simulink model "quad_with_sensor_fusion_discrete"  (R2022b)
settings: Solver=FixedStepDiscrete  StartTime=0.0  StopTime=120  FixedStep=0.005  RelTol=1e-3
values from neighbouring files (symbols this model uses):
  Ixc = 9373.661914436/1e6    (= 0.00937366191444)    [ParamsInit_test.m]
  Iyc = 11755.067703159/1e6    (= 0.0117550677032)    [ParamsInit_test.m]
  Izc = 17533.553367555/1e6    (= 0.0175335533676)    [ParamsInit_test.m]
  kd_h = damp_ratio_h*2*sqrt(kp_h*Vehicle.Airframe.mass)    [ParamsInit_test.m]
  kd_phi = damp_ratio_phi*2*sqrt(kp_phi*Ixc)    [ParamsInit_test.m]
  kd_theta = damp_ratio_theta*2*sqrt(kp_theta*Iyc)    [ParamsInit_test.m]
  kd_yaw = damp_ratio_yaw*2*sqrt(kp_yaw*Izc)    [ParamsInit_test.m]
  kp_h = omega_n_h^2*Vehicle.Airframe.mass    [ParamsInit_test.m]
  kp_phi = omega_n_phi^2*Ixc    (= 0.937366191444)    [ParamsInit_test.m]
  kp_position = 0.1    [ParamsInit_test.m]
  kp_theta = omega_n_theta^2*Iyc    (= 1.17550677032)    [ParamsInit_test.m]
  kp_vx = 0.25    [ParamsInit_test.m]
  kp_vy = 0.25    [ParamsInit_test.m]
  kp_yaw = omega_n_yaw^2*Izc    (= 0.0175335533676)    [ParamsInit_test.m]
undefined symbols (not defined in the file or in its folder): DiscIntNeverNeededParam, Vehicle
libraries: simulink x3, aerolibconvert2 x2, mspfiltlib x1, sensorinslib x1, aerolibasang x1, sharedtransform x1, mspsensorlib x1, sensorgpslib x1, aerolibanimutils x1, uavutilslib x1
(part 1 of 2)
settings Model: Creator=gaowe  LastModifiedBy=GMS
settings ModelReferenceCC: EnableRefExpFcnMdlSchedulingChecks=on
settings RTWCC: DLArmComputeVersion=19.05

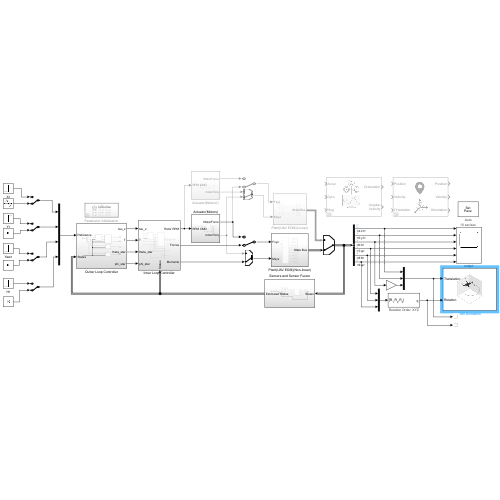
[thumbnail: Simulink's stored preview of the top-level diagram]
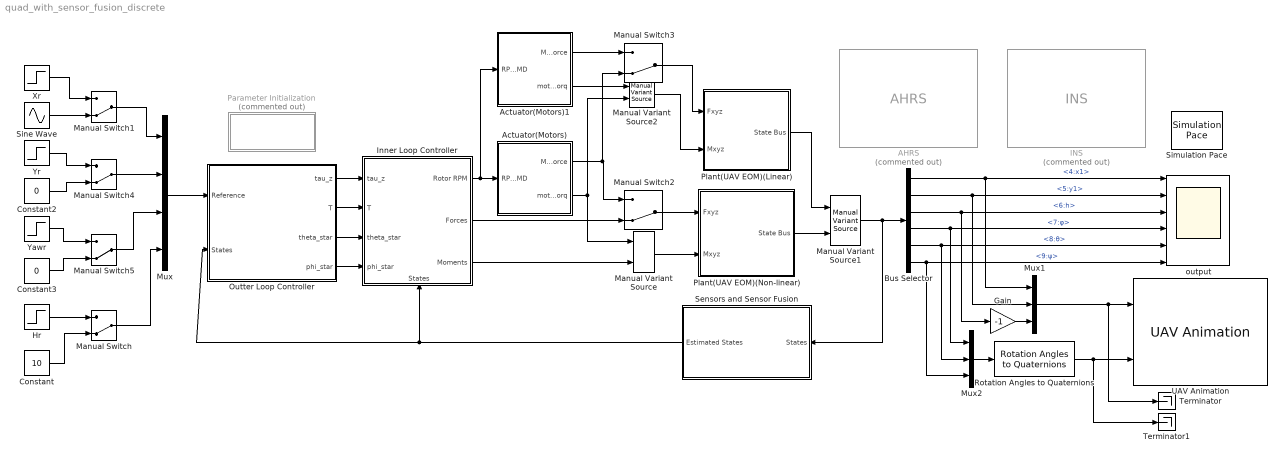
== system quad_with_sensor_fusion_discrete ==
  AHRS : mspfiltlib/AHRS  Commented=on  DispRefFrame=NED  DecimationFactor=1  InitialProcessNoise=ahrsfilter.defaultProcessNoise  OrientationFormat=quaternion  SimulateUsing=Interpreted execution  AccelerometerNoise=0.0001924722  GyroscopeNoise=9.1385e-5  MagnetometerNoise=0.1  GyroscopeDriftNoise=3.0462e-13  LinearAccelerationNoise=0.0096236100000000012  MagneticDisturbanceNoise=0.5  LinearAccelerationDecayFactor=0.5  MagneticDisturbanceDecayFactor=0.5  ExpectedMagneticFieldStrength=50
  Actuator(Motors) : Subsystem
  Actuator(Motors)1 : Subsystem
  Bus Selector : BusSelector  OutputSignals=4:x1,5:y1,6:h,7:φ,8:θ,9:ψ
  Constant : Constant  Value=10  SampleTime=0.005
  Constant2 : Constant  Value=0  SampleTime=0.005
  Constant3 : Constant  Value=0  SampleTime=0.005
  Gain : Gain  Gain=-1
  Hr : Step  Time=0  After=20  SampleTime=0.005
  INS : sensorinslib/INS  Commented=on  MountingLocation=[0 0 0]  RollAccuracy=0.2  PitchAccuracy=0.2  YawAccuracy=1  PositionAccuracy=1  VelocityAccuracy=0.05  UseAccelAndAngVel=off  AccelerationAccuracy=0  AngularVelocityAccuracy=0  TimeInput=off  PositionErrorFactor=[0 0 0]  SeedDouble=67  SimulateUsing=Interpreted execution
      settings: LibrarySourceBlock=uavsimlib/INS
  Inner Loop Controller : Subsystem
      settings: PortSchema="{\"entries\":[{\"content\":{\"sides\":[{\"content\":{\"connectorIds\":[\"In1\",\"In2\",\"In3\",\"In4\"]},\"type\":\"ConnectorPlacement.EquallySpacedRectSide\",\"uuid\":\"3024e14a-e42b-4ece-95b6-8188e577f7ea\"},{\"content\":{\"connectorIds\":[\"Out1\",\"Out2\",\"Out3\"],\"side\":\"RIGHT\"},\"type\":\"ConnectorPlacement.EquallySpacedRectSide\",\"uuid\":\"28791f10-00d9-435c-9b3a-62150bd300bc\"},{\"content\":{\"connectorIds\":[],\"side\":\"TOP\"},\"type\":\"ConnectorPlacement.EquallySpacedRectSide\",\"uuid\":\"5a81466d-668a-47df-a46c-2854fa138474\"},{\"content\":{\"connectorIds\":[\"In5\"],\"side\":\"BOTTOM\"},\"type\":\"ConnectorPlacement.EquallySpacedRectSide\",\"uuid\":\"dc01fcce-ea7b-43d7-98f8-2115160ba315\"}]},\"type\":\"ConnectorPlacement.EquallySpacedConnector\",\"uuid\":\"802a1a82-5ed7-4d3a-8fbf-5749d0aa0952\"}],\"packageUris\":[\"http://schema.mathworks.com/mf0/Connector/R2020b\"],\"version\":\"1.0\"}"
  Manual Variant Source : simulink/Signal Routing/Manual Variant Source  NumChoices=2  LabelModeActiveChoice=V_2
  Manual Variant Source1 : simulink/Signal Routing/Manual Variant Source  NumChoices=2  LabelModeActiveChoice=V_2
  Manual Variant Source2 : simulink/Signal Routing/Manual Variant Source  NumChoices=2  LabelModeActiveChoice=V_2
  Manual Switch{,1..5} (6 alike) : ManualSwitch  CurrentSetting=0
  Mux : Mux
  Mux1 : Mux  Inputs=3
  Mux2 : Mux  Inputs=3
  Outter Loop Controller : Subsystem
  Parameter Initialization : Subsystem  Commented=on  TreatAsAtomicUnit=on
  Plant(UAV EOM)(Linear) : Subsystem
  Plant(UAV EOM)(Non-linear) : Subsystem
  Rotation Angles to Quaternions : sharedtransform/Rotation Angles to Quaternions  rotationOrder=XYZ  aMode=aMode
  Sensors and Sensor Fusion : Subsystem
  Simulation Pace : aerolibanimutils/Simulation Pace  SimulationPace=10  SleepMode=Auto  OutputPaceError=off  SampleTime=1/100
  Sine Wave : Sin  SineType=Sample based  Amplitude=10  Frequency=2*pi/60  Samples=12000  SampleTime=0.005
  Terminator : Terminator
  Terminator1 : Terminator
  UAV Animation : uavutilslib/UAV Animation  UAVType=Multirotor  UAVSize=1  InertialZDirection=Down  SampleTime=0.005
  Xr : Step  Time=0  After=10  SampleTime=0.005
  Yawr : Step  Time=0  After=pi/2  SampleTime=0.005
  Yr : Step  Time=0  After=10  SampleTime=0.005
  output : Scope  NumInputPorts=6
  wires:
  Manual Variant Source1/1 -> Sensors and Sensor Fusion/1(States), Bus Selector/1
  Mux/1 -> Outter Loop Controller/1(Reference)
  Manual Switch1/1 -> Mux/1
  Constant2/1 -> Manual Switch4/2
  Yawr/1 -> Manual Switch5/1
  Hr/1 -> Manual Switch/1
  Outter Loop Controller/3(theta_star) -> Inner Loop Controller/3(theta_star)
  Outter Loop Controller/1(tau_z) -> Inner Loop Controller/1(tau_z)
  Outter Loop Controller/2(T) -> Inner Loop Controller/2(T)
  Outter Loop Controller/4(phi_star) -> Inner Loop Controller/4(phi_star)
  Inner Loop Controller/1(Rotor RPM) -> Actuator(Motors)1/1(RPM CMD), Actuator(Motors)/1(RPM CMD)
  Actuator(Motors)/1(MotorForce) -> Manual Switch3/2, Manual Switch2/1
  Actuator(Motors)/2(motorTorq) -> Manual Variant Source2/2, Manual Variant Source/1
  Bus Selector/1 -> Mux1/1, output/1  "<4:x1>"
  Bus Selector/2 -> Mux1/2, output/2  "<5:y1>"
  Bus Selector/3 -> Gain/1, output/3  "<6:h>"
  Bus Selector/4 -> Mux2/1, output/4  "<7:φ>"
  Bus Selector/5 -> Mux2/2, output/5  "<8:θ>"
  Bus Selector/6 -> Mux2/3, output/6  "<9:ψ>"
  Manual Switch/1 -> Mux/4
  Constant/1 -> Manual Switch/2
  Sine Wave/1 -> Manual Switch1/2
  Xr/1 -> Manual Switch1/1
  Inner Loop Controller/2(Forces) -> Manual Switch2/2
  Inner Loop Controller/3(Moments) -> Manual Variant Source/2
  Plant(UAV EOM)(Linear)/1(State Bus) -> Manual Variant Source1/1
  Manual Variant Source/1 -> Plant(UAV EOM)(Non-linear)/2(Mxyz)
  Manual Switch2/1 -> Plant(UAV EOM)(Non-linear)/1(Fxyz)
  Plant(UAV EOM)(Non-linear)/1(State Bus) -> Manual Variant Source1/2
  Actuator(Motors)1/1(MotorForce) -> Manual Switch3/1
  Actuator(Motors)1/2(motorTorq) -> Manual Variant Source2/1
  Manual Switch3/1 -> Plant(UAV EOM)(Linear)/1(Fxyz)
  Manual Variant Source2/1 -> Plant(UAV EOM)(Linear)/2(Mxyz)
  Manual Switch4/1 -> Mux/2
  Yr/1 -> Manual Switch4/1
  Constant3/1 -> Manual Switch5/2
  Manual Switch5/1 -> Mux/3
  Mux1/1 -> Terminator/1, UAV Animation/1
  Rotation Angles to Quaternions/1 -> Terminator1/1, UAV Animation/2
  Mux2/1 -> Rotation Angles to Quaternions/1
  Gain/1 -> Mux1/3
  Sensors and Sensor Fusion/1(Estimated States) -> Outter Loop Controller/2(States), Inner Loop Controller/5(States)

== system quad_with_sensor_fusion_discrete/Actuator(Motors) ==
  RPM CMD : Inport
  -k_T : Gain  Gain=-1.097e-5
  D4 : Constant  Value=0  SampleTime=0.005
  D5 : Constant  Value=0  SampleTime=0.005
  Mux4 : Mux  Inputs=3
  Propeller Model : MATLAB Function  TreatAsAtomicUnit=on
  Square : Math  Operator=square
  Sum of Elements : Sum  Inputs=+
  k_tau : Gain  Gain=1.779e-07
  rpm2rads : Gain  Gain=pi/30
  MotorForce : Outport
  motorTorq : Outport  Port=2
  wires:
  k_tau/1 -> motorTorq/1
  Mux4/1 -> MotorForce/1
  Sum of Elements/1 -> Mux4/3
  -k_T/1 -> Sum of Elements/1
  Square/1 -> -k_T/1, Propeller Model/1(F)
  Propeller Model/1(Mb_xy) -> k_tau/1
  D4/1 -> Mux4/1
  D5/1 -> Mux4/2
  RPM CMD/1 -> rpm2rads/1
  rpm2rads/1 -> Square/1

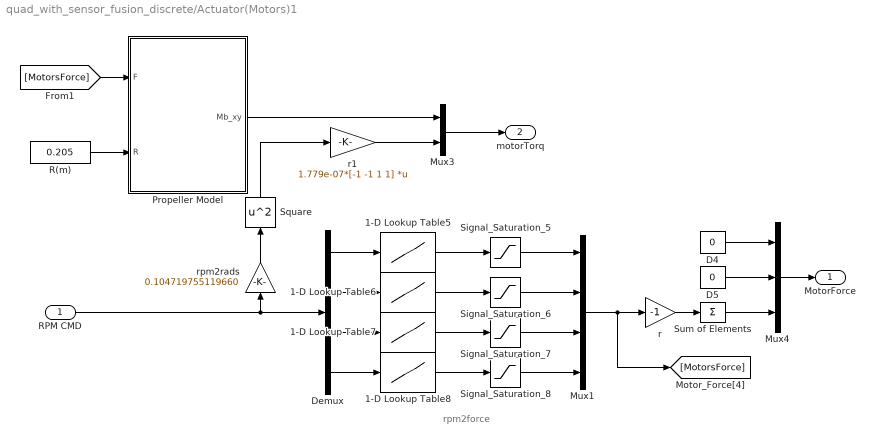
== system quad_with_sensor_fusion_discrete/Actuator(Motors)1 ==
  note: rpm2force
  RPM CMD : Inport
  1-D Lookup Table5 : Lookup_n-D  NumberOfTableDimensions=1  BreakpointsForDimension1=|  BeginIndexSearchUsingPreviousIndexResult=on  Table=|  InternalRulePriority=Speed  RndMeth=Simplest
      BreakpointsForDimension1=|
      | [2847
      | 3689
      | 4585
      | 5400
      | 6400
      | 7000
      | 7800
      | 8222
      | 9300
      | 10700]
      Table=|
      | [0.6664
      | 1.4308
      | 2.3422
      | 3.3418
      | 4.9098
      | 5.929
      | 7.399
      | 7.6244
      | 10.976
      | 13.72]
  1-D Lookup Table6 : Lookup_n-D  NumberOfTableDimensions=1  BreakpointsForDimension1=|  BeginIndexSearchUsingPreviousIndexResult=on  Table=|  InternalRulePriority=Speed  RndMeth=Simplest
      BreakpointsForDimension1=|
      | [2847
      | 3689
      | 4585
      | 5400
      | 6400
      | 7000
      | 7800
      | 8222
      | 9300
      | 10700]
      Table=|
      | [0.6664
      | 1.4308
      | 2.3422
      | 3.3418
      | 4.9098
      | 5.929
      | 7.399
      | 7.6244
      | 10.976
      | 13.72]
  1-D Lookup Table7 : Lookup_n-D  NumberOfTableDimensions=1  BreakpointsForDimension1=|  BeginIndexSearchUsingPreviousIndexResult=on  Table=|  InternalRulePriority=Speed  RndMeth=Simplest
      BreakpointsForDimension1=|
      | [2847
      | 3689
      | 4585
      | 5400
      | 6400
      | 7000
      | 7800
      | 8222
      | 9300
      | 10700]
      Table=|
      | [0.6664
      | 1.4308
      | 2.3422
      | 3.3418
      | 4.9098
      | 5.929
      | 7.399
      | 7.6244
      | 10.976
      | 13.72]
  1-D Lookup Table8 : Lookup_n-D  NumberOfTableDimensions=1  BreakpointsForDimension1=|  BeginIndexSearchUsingPreviousIndexResult=on  Table=|  InternalRulePriority=Speed  RndMeth=Simplest
      BreakpointsForDimension1=|
      | [2847
      | 3689
      | 4585
      | 5400
      | 6400
      | 7000
      | 7800
      | 8222
      | 9300
      | 10700]
      Table=|
      | [0.6664
      | 1.4308
      | 2.3422
      | 3.3418
      | 4.9098
      | 5.929
      | 7.399
      | 7.6244
      | 10.976
      | 13.72]
  D4 : Constant  Value=0
  D5 : Constant  Value=0
  Demux : Demux
  Mux1 : Mux
  Mux3 : Mux  Inputs=[2 1]
  Mux4 : Mux  Inputs=3
  Propeller Model : MATLAB Function  TreatAsAtomicUnit=on
  R(m) : Constant  Value=0.205
  Signal_Saturation_{5..8} (4 alike) : Saturate  UpperLimit=1.4*9.8  LowerLimit=0
  Square : Math  Operator=square
  Sum of Elements : Sum  Inputs=+
  r : Gain  Gain=-1
  r1 : Gain  Gain=1.779e-07*[-1 -1 1 1]  Multiplication=Matrix(K*u)
  rpm2rads : Gain  Gain=0.104719755119660
  MotorForce : Outport
  motorTorq : Outport  Port=2
  wires:
  Signal_Saturation_6/1 -> Mux1/2
  1-D Lookup Table7/1 -> Signal_Saturation_7/1
  Mux3/1 -> motorTorq/1
  1-D Lookup Table6/1 -> Signal_Saturation_6/1
  Mux4/1 -> MotorForce/1
  r1/1 -> Mux3/2
  Sum of Elements/1 -> Mux4/3
  r/1 -> Sum of Elements/1
  Mux1/1 -> [MotorsForce], r/1
  Demux/1 -> 1-D Lookup Table5/1
  Square/1 -> r1/1
  1-D Lookup Table5/1 -> Signal_Saturation_5/1
  Demux/3 -> 1-D Lookup Table7/1
  Signal_Saturation_5/1 -> Mux1/1
  1-D Lookup Table8/1 -> Signal_Saturation_8/1
  [MotorsForce] -> Propeller Model/1(F)
  Demux/4 -> 1-D Lookup Table8/1
  Demux/2 -> 1-D Lookup Table6/1
  Signal_Saturation_7/1 -> Mux1/3
  Propeller Model/1(Mb_xy) -> Mux3/1
  Signal_Saturation_8/1 -> Mux1/4
  R(m)/1 -> Propeller Model/2(R)
  D4/1 -> Mux4/1
  D5/1 -> Mux4/2
  RPM CMD/1 -> Demux/1, rpm2rads/1
  rpm2rads/1 -> Square/1

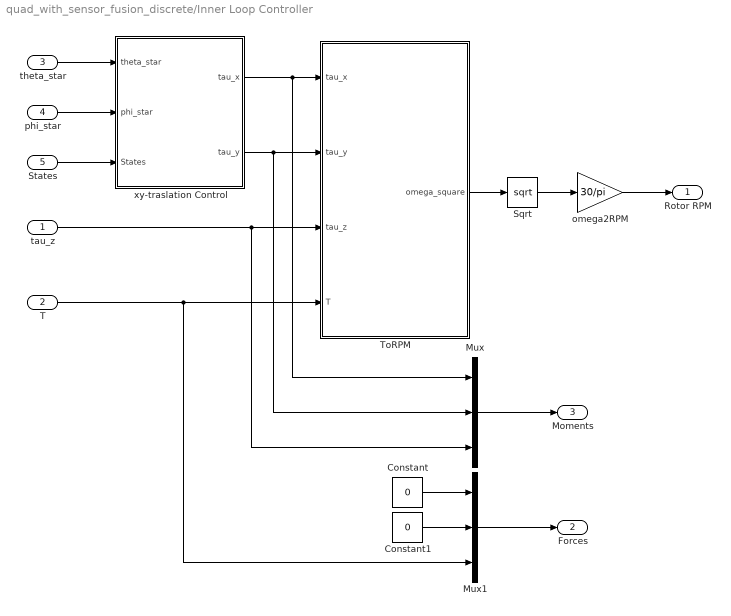
== system quad_with_sensor_fusion_discrete/Inner Loop Controller ==
  tau_z : Inport
  T : Inport  Port=2
  theta_star : Inport  Port=3
  phi_star : Inport  Port=4
  States : Inport  Port=5
  Constant : Constant  Value=0  SampleTime=0.005
  Constant1 : Constant  Value=0  SampleTime=0.005
  Mux : Mux  Inputs=3
  Mux1 : Mux  Inputs=3
  Sqrt : Sqrt
  ToRPM : MATLAB Function  TreatAsAtomicUnit=on
  omega2RPM : Gain  Gain=30/pi
  xy-traslation Control : Subsystem
  Rotor RPM : Outport
  Forces : Outport  Port=2
  Moments : Outport  Port=3
  wires:
  theta_star/1 -> xy-traslation Control/1(theta_star)
  States/1 -> xy-traslation Control/3(States)
  phi_star/1 -> xy-traslation Control/2(phi_star)
  tau_z/1 -> Mux/3, ToRPM/3(tau_z)
  xy-traslation Control/2(tau_y) -> Mux/2, ToRPM/2(tau_y)
  xy-traslation Control/1(tau_x) -> Mux/1, ToRPM/1(tau_x)
  Sqrt/1 -> omega2RPM/1
  omega2RPM/1 -> Rotor RPM/1
  ToRPM/1(omega_square) -> Sqrt/1
  Mux/1 -> Moments/1
  Constant/1 -> Mux1/1
  Constant1/1 -> Mux1/2
  Mux1/1 -> Forces/1
  T/1 -> Mux1/3, ToRPM/4(T)

== system quad_with_sensor_fusion_discrete/Outter Loop Controller ==
  Reference : Inport
  States : Inport  Port=2
  Demux : Demux
  Height Control : Subsystem
  Position Control : Subsystem
  Velocity Control : Subsystem
  Yaw Control : Subsystem
  tau_z : Outport
  T : Outport  Port=2
  theta_star : Outport  Port=3
  phi_star : Outport  Port=4
  wires:
  Reference/1 -> Demux/1
  States/1 -> Position Control/3(States), Velocity Control/3(States), Yaw Control/2(States), Height Control/2(States)
  Velocity Control/1(theta_star) -> theta_star/1
  Demux/4 -> Height Control/1(Hr)  "Hr"
  Demux/3 -> Yaw Control/1(Yawr)  "Yawr"
  Demux/2 -> Position Control/2(yr)  "Yr"
  Demux/1 -> Position Control/1(xr)  "Xr"
  Height Control/1(T) -> T/1
  Yaw Control/1(tau_z) -> tau_z/1
  Velocity Control/2(phi_star) -> phi_star/1
  Position Control/1(vxr) -> Velocity Control/1(vxr)
  Position Control/2(vyr) -> Velocity Control/2(vyr)

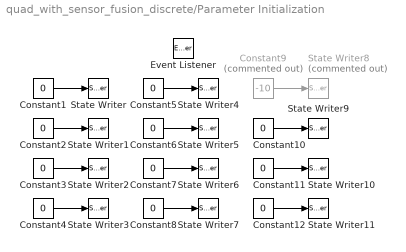
== system quad_with_sensor_fusion_discrete/Parameter Initialization ==
  Constant{1..8,10..12} (11 alike) : Constant  Value=0
  Constant9 : Constant  Commented=on  Value=-10
  Event Listener : EventListener  DisableCoverage=on  EventName=reset
  State Writer{,1..7,9..11} (11 alike) : StateWriter
  State Writer8 : StateWriter  Commented=on
  wires:
  Constant1/1 -> State Writer/1
  Constant2/1 -> State Writer1/1
  Constant4/1 -> State Writer3/1
  Constant3/1 -> State Writer2/1
  Constant6/1 -> State Writer5/1
  Constant7/1 -> State Writer6/1
  Constant5/1 -> State Writer4/1
  Constant8/1 -> State Writer7/1
  Constant10/1 -> State Writer9/1
  Constant11/1 -> State Writer10/1
  Constant9/1 -> State Writer8/1
  Constant12/1 -> State Writer11/1

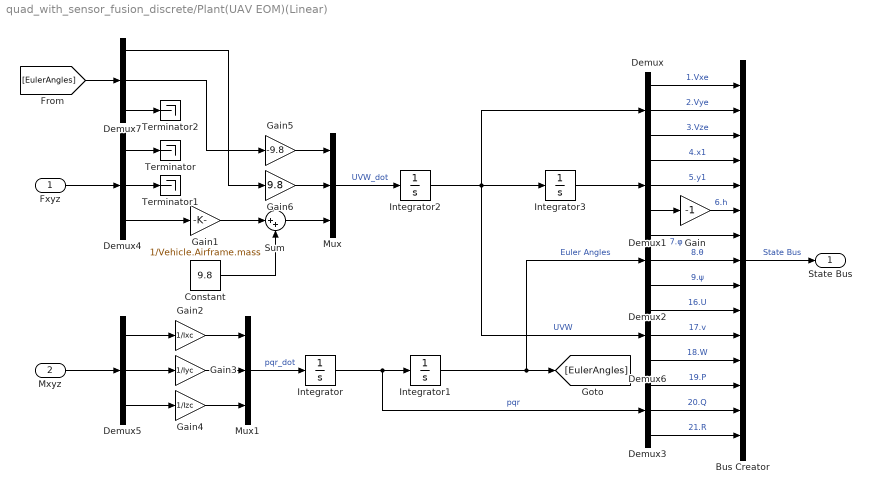
== system quad_with_sensor_fusion_discrete/Plant(UAV EOM)(Linear) ==
  Fxyz : Inport
  Mxyz : Inport  Port=2
  Bus Creator : BusCreator  Inputs=15
  Constant : Constant  Value=9.8
  Demux{,1..7} (8 alike) : Demux  Outputs=3
  Gain : Gain  Gain=-1
  Gain1 : Gain  Gain=1/Vehicle.Airframe.mass
  Gain2 : Gain  Gain=1/Ixc
  Gain3 : Gain  Gain=1/Iyc
  Gain4 : Gain  Gain=1/Izc
  Gain5 : Gain  Gain=-9.8
  Gain6 : Gain  Gain=9.8
  Integrator : Integrator  InitialCondition=[0,0,0]
  Integrator1 : Integrator  InitialCondition=[0,0,0]
  Integrator2 : Integrator  InitialCondition=[0,0,0]
  Integrator3 : Integrator  InitialCondition=[0,0,-10]
  Mux : Mux  Inputs=3
  Mux1 : Mux  Inputs=3
  Sum : Sum  Inputs=|++
  Terminator : Terminator
  Terminator1 : Terminator
  Terminator2 : Terminator
  State Bus : Outport
  wires:
  Gain/1 -> Bus Creator/6  "6.h"
  Demux/1 -> Bus Creator/1  "1.Vxe"
  Demux6/2 -> Bus Creator/11  "17.v"
  Demux3/3 -> Bus Creator/15  "21.R"
  Demux3/1 -> Bus Creator/13  "19.P"
  Demux6/1 -> Bus Creator/10  "16.U"
  Demux2/2 -> Bus Creator/8  "8.θ"
  Demux2/1 -> Bus Creator/7  "7.φ"
  Demux1/3 -> Gain/1
  Demux2/3 -> Bus Creator/9  "9.ψ"
  Demux1/2 -> Bus Creator/5  "5.y1"
  Demux3/2 -> Bus Creator/14  "20.Q"
  Demux6/3 -> Bus Creator/12  "18.W"
  Demux/3 -> Bus Creator/3  "3.Vze"
  Demux1/1 -> Bus Creator/4  "4.x1"
  Demux/2 -> Bus Creator/2  "2.Vye"
  Bus Creator/1 -> State Bus/1  "State Bus"
  Fxyz/1 -> Demux4/1
  Mxyz/1 -> Demux5/1
  Demux4/1 -> Terminator/1
  Demux4/2 -> Terminator1/1
  Demux4/3 -> Gain1/1
  Gain1/1 -> Sum/1
  Demux5/2 -> Gain3/1
  Demux5/1 -> Gain2/1
  Demux5/3 -> Gain4/1
  Mux1/1 -> Integrator/1  "pqr_dot"
  Gain3/1 -> Mux1/2
  Gain2/1 -> Mux1/1
  Gain4/1 -> Mux1/3
  Integrator/1 -> Demux3/1, Integrator1/1  "pqr"
  Integrator1/1 -> [EulerAngles], Demux2/1  "Euler Angles"
  Gain5/1 -> Mux/1
  [EulerAngles] -> Demux7/1
  Demux7/1 -> Gain6/1
  Demux7/2 -> Gain5/1
  Gain6/1 -> Mux/2
  Demux7/3 -> Terminator2/1
  Mux/1 -> Integrator2/1  "UVW_dot"
  Integrator2/1 -> Demux/1, Integrator3/1, Demux6/1  "UVW"
  Integrator3/1 -> Demux1/1
  Constant/1 -> Sum/2
  Sum/1 -> Mux/3

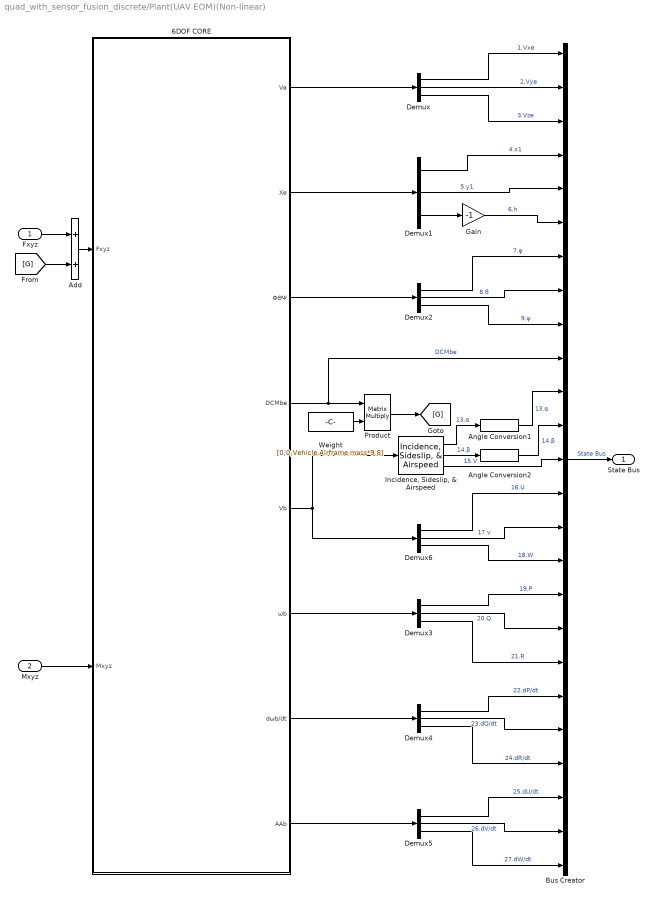
== system quad_with_sensor_fusion_discrete/Plant(UAV EOM)(Non-linear) ==
  Fxyz : Inport
  Mxyz : Inport  Port=2
  6DOF CORE : Subsystem
  Add : Sum
  Angle Conversion1 : aerolibconvert2/Angle Conversion  IU=rad  OU=deg
  Angle Conversion2 : aerolibconvert2/Angle Conversion  IU=rad  OU=deg
  Bus Creator : BusCreator  Inputs=25
  Demux{,1..6} (7 alike) : Demux  Outputs=3
  Gain : Gain  Gain=-1
  "Incidence, Sideslip, & Airspeed" : aerolibasang/Incidence, Sideslip, & Airspeed
  Product : Product  Multiplication=Matrix(*)
  Weight : Constant  Value=[0;0;Vehicle.Airframe.mass*9.8]  VectorParams1D=off  SampleTime=0.005
  State Bus : Outport
  wires:
  Gain/1 -> Bus Creator/6  "6.h"
  6DOF CORE/5(Vb) -> "Incidence, Sideslip, & Airspeed"/1, Demux6/1
  6DOF CORE/1(Ve) -> Demux/1
  Demux/1 -> Bus Creator/1  "1.Vxe"
  Demux6/2 -> Bus Creator/15  "17.v"
  6DOF CORE/3(ΦΘΨ) -> Demux2/1
  Demux3/3 -> Bus Creator/19  "21.R"
  Demux5/3 -> Bus Creator/25  "27.dW/dt"
  Demux4/3 -> Bus Creator/22  "24.dR/dt"
  "Incidence, Sideslip, & Airspeed"/3 -> Bus Creator/13  "15.V"
  Demux3/1 -> Bus Creator/17  "19.P"
  Demux6/1 -> Bus Creator/14  "16.U"
  6DOF CORE/7(dωb/dt) -> Demux4/1
  Demux2/2 -> Bus Creator/8  "8.θ"
  Demux2/1 -> Bus Creator/7  "7.φ"
  "Incidence, Sideslip, & Airspeed"/1 -> Angle Conversion1/1  "13.α"
  6DOF CORE/6(ωb) -> Demux3/1
  Demux1/3 -> Gain/1
  6DOF CORE/2(Xe) -> Demux1/1
  Demux2/3 -> Bus Creator/9  "9.ψ"
  Demux4/2 -> Bus Creator/21  "23.dQ/dt"
  Demux5/2 -> Bus Creator/24  "26.dV/dt"
  Demux1/2 -> Bus Creator/5  "5.y1"
  Demux3/2 -> Bus Creator/18  "20.Q"
  Angle Conversion2/1 -> Bus Creator/12  "14.β"
  Demux5/1 -> Bus Creator/23  "25.dU/dt"
  Demux6/3 -> Bus Creator/16  "18.W"
  6DOF CORE/8(AAb) -> Demux5/1
  Demux4/1 -> Bus Creator/20  "22.dP/dt"
  Angle Conversion1/1 -> Bus Creator/11  "13.α"
  Demux/3 -> Bus Creator/3  "3.Vze"
  "Incidence, Sideslip, & Airspeed"/2 -> Angle Conversion2/1  "14.β"
  Demux1/1 -> Bus Creator/4  "4.x1"
  Demux/2 -> Bus Creator/2  "2.Vye"
  Bus Creator/1 -> State Bus/1  "State Bus"
  Fxyz/1 -> Add/1
  Mxyz/1 -> 6DOF CORE/2(Mxyz)
  Product/1 -> [G]
  Weight/1 -> Product/2
  6DOF CORE/4(DCMbe) -> Bus Creator/10, Product/1  "DCMbe"
  [G] -> Add/2
  Add/1 -> 6DOF CORE/1(Fxyz)

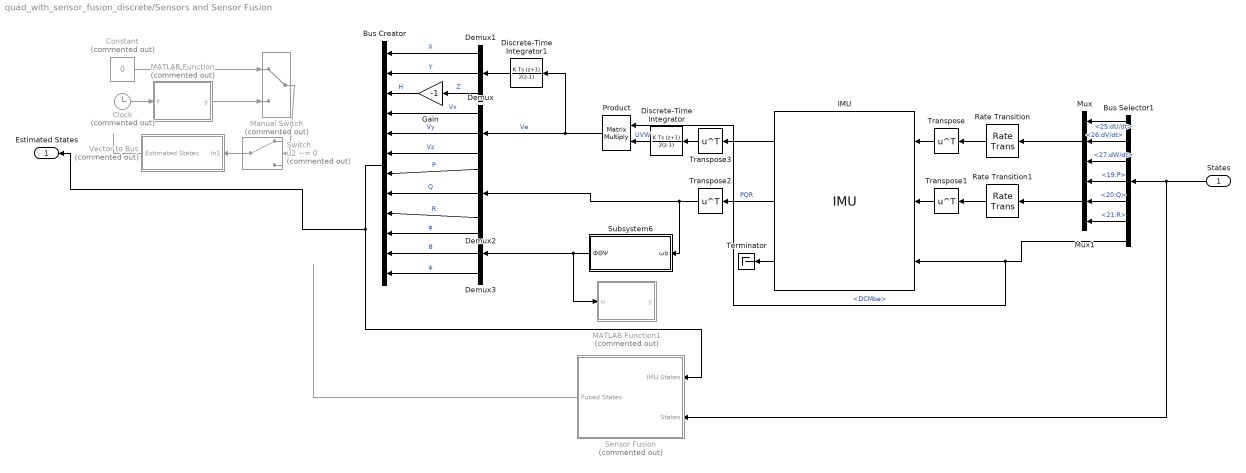
== system quad_with_sensor_fusion_discrete/Sensors and Sensor Fusion ==
  States : Inport
  Bus Creator : BusCreator  Inputs=12
  Bus Selector1 : BusSelector  OutputSignals=25:dU/dt,26:dV/dt,27:dW/dt,19:P,20:Q,21:R,DCMbe
  Clock : Clock  Commented=on
  Constant : Constant  Commented=on  Value=0  SampleTime=0.005
  Demux{,1..3} (4 alike) : Demux  Outputs=3
  Discrete-Time Integrator : DiscreteIntegrator  IntegratorMethod=Integration: Trapezoidal  SampleTime=0.005  ICPrevOutput=DiscIntNeverNeededParam  ICPrevScaledInput=DiscIntNeverNeededParam
  Discrete-Time Integrator1 : DiscreteIntegrator  IntegratorMethod=Integration: Trapezoidal  SampleTime=0.005  ICPrevOutput=DiscIntNeverNeededParam  ICPrevScaledInput=DiscIntNeverNeededParam
  Gain : Gain  Gain=-1
  IMU : mspsensorlib/IMU  DispRefFrame=NED  Temperature=25  MagneticFieldNED=[ 27.5550, -2.4169, -16.0849 ]  MagneticFieldENU=[ -2.4169, 27.5550, 16.0849 ]  SeedDouble=67  SimulateUsing=Interpreted execution  AccelParamsMeasurementRange=19.613  AccelParamsResolution=0.0023928  AccelParamsConstantBias=[ 0, 0, 0 ]  AccelParamsAxesMisalignment=[0 0 0]  AccelParamsNoiseDensity=0.01*ones(1,3)  AccelParamsBiasInstability=[ 0, 0, 0 ]  AccelParamsRandomWalk=[ 0, 0, 0 ]  AccelParamsTemperatureBias=[ 0, 0, 0 ]  AccelParamsTemperatureScaleFactor=[ 0, 0, 0 ]  GyroParamsMeasurementRange=4.3633  GyroParamsResolution=0.0011  GyroParamsConstantBias=[ 0, 0, 0 ]  GyroParamsAxesMisalignment=0  GyroParamsAccelerationBias=[ 0, 0, 0 ]  GyroParamsNoiseDensity=1e-3*ones(1,3)  GyroParamsBiasInstability=[ 0, 0, 0 ]  GyroParamsRandomWalk=[ 0, 0, 0 ]  GyroParamsTemperatureBias=[ 0, 0, 0 ]  GyroParamsTemperatureScaleFactor=[ 0, 0, 0 ]  MagParamsMeasurementRange=1000  MagParamsResolution=0.1  MagParamsConstantBias=[ 0, 0, 0 ]  MagParamsAxesMisalignment=[0 0 0]  MagParamsNoiseDensity=[0.0424 0.0424 0.0424]  MagParamsBiasInstability=[ 0, 0, 0 ]  MagParamsRandomWalk=[ 0, 0, 0 ]  MagParamsTemperatureBias=[ 0, 0, 0 ]  MagParamsTemperatureScaleFactor=[ 0, 0, 0 ]
  MATLAB Function : MATLAB Function  Commented=on  TreatAsAtomicUnit=on
  MATLAB Function1 : MATLAB Function  Commented=on  TreatAsAtomicUnit=on
  Manual Switch : ManualSwitch  Commented=on
  Mux : Mux  Inputs=3
  Mux1 : Mux  Inputs=3
  Product : Product  Multiplication=Matrix(*)
  Rate Transition : RateTransition
  Rate Transition1 : RateTransition
  Sensor Fusion : Subsystem  Commented=on
  Subsystem6 : Subsystem
  Switch : Switch  Commented=on  Criteria=u2 ~= 0  SaturateOnIntegerOverflow=off  InputSameDT=off
  Terminator : Terminator
  Transpose{,1..3} (4 alike) : Math  Operator=transpose
  Vector to Bus : Subsystem  Commented=on
  Estimated States : Outport
  wires:
  Bus Creator/1 -> Estimated States/1, Sensor Fusion/1(IMU States)
  States/1 -> Sensor Fusion/2(States), Bus Selector1/1
  Subsystem6/1(ΦΘΨ) -> MATLAB Function1/1(u), Demux3/1
  Bus Selector1/4 -> Mux1/1  "<19:P>"
  Bus Selector1/5 -> Mux1/2  "<20:Q>"
  Bus Selector1/6 -> Mux1/3  "<21:R>"
  Bus Selector1/1 -> Mux/1  "<25:dU/dt>"
  Bus Selector1/2 -> Mux/2  "<26:dV/dt>"
  Bus Selector1/3 -> Mux/3  "<27:dW/dt>"
  Clock/1 -> MATLAB Function/1(t)
  MATLAB Function/1(y) -> Manual Switch/2
  IMU/3 -> Terminator/1
  IMU/1 -> Transpose3/1
  IMU/2 -> Transpose2/1  "PQR"
  Discrete-Time Integrator/1 -> Product/2  "UVW"
  Product/1 -> Discrete-Time Integrator1/1, Demux/1  "Ve"
  Demux/1 -> Bus Creator/4  "Vx"
  Demux/2 -> Bus Creator/5  "Vy"
  Demux/3 -> Bus Creator/6  "Vz"
  Discrete-Time Integrator1/1 -> Demux1/1
  Demux1/1 -> Bus Creator/1  "X"
  Demux1/2 -> Bus Creator/2  "Y"
  Demux1/3 -> Gain/1  "Z"
  Gain/1 -> Bus Creator/3  "H"
  Demux2/1 -> Bus Creator/7  "P"
  Demux2/2 -> Bus Creator/8  "Q"
  Demux2/3 -> Bus Creator/9  "R"
  Demux3/1 -> Bus Creator/10  "φ"
  Demux3/2 -> Bus Creator/11  "θ"
  Demux3/3 -> Bus Creator/12  "ψ"
  Bus Selector1/7 -> Product/1, IMU/3  "<DCMbe>"
  Sensor Fusion/1(Fused States) -> ?
  Vector to Bus/1(Estimated States) -> ?
  Constant/1 -> Manual Switch/1
  Manual Switch/1 -> Switch/2
  Switch/1 -> Vector to Bus/1(In1)
  Transpose/1 -> IMU/1
  Transpose1/1 -> IMU/2
  Mux/1 -> Rate Transition/1
  Mux1/1 -> Rate Transition1/1
  Rate Transition/1 -> Transpose/1
  Rate Transition1/1 -> Transpose1/1
  Transpose2/1 -> Subsystem6/1(ωb), Demux2/1
  Transpose3/1 -> Discrete-Time Integrator/1

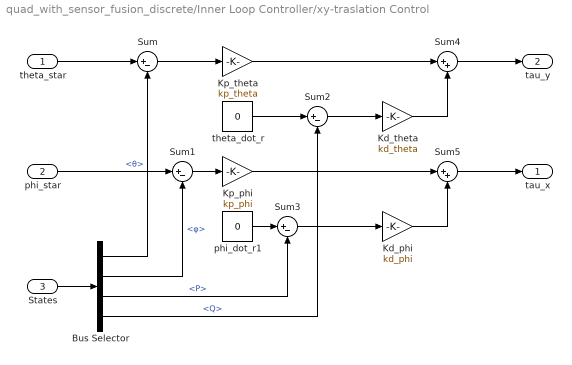
== system quad_with_sensor_fusion_discrete/Inner Loop Controller/xy-traslation Control ==
  theta_star : Inport
  phi_star : Inport  Port=2
  States : Inport  Port=3
  Bus Selector : BusSelector  OutputSignals=θ,φ,P,Q
  Kd_phi : Gain  Gain=kd_phi
  Kd_theta : Gain  Gain=kd_theta
  Kp_phi : Gain  Gain=kp_phi
  Kp_theta : Gain  Gain=kp_theta
  Sum{,1..3} (4 alike) : Sum  Inputs=|+-
  Sum4 : Sum  Inputs=|++
  Sum5 : Sum  Inputs=|++
  phi_dot_r1 : Constant  Value=0  SampleTime=0.005
  theta_dot_r : Constant  Value=0  SampleTime=0.005
  tau_x : Outport
  tau_y : Outport  Port=2
  wires:
  theta_star/1 -> Sum/1
  States/1 -> Bus Selector/1
  Bus Selector/1 -> Sum/2  "<θ>"
  phi_star/1 -> Sum1/1
  Bus Selector/2 -> Sum1/2  "<φ>"
  Sum/1 -> Kp_theta/1
  Sum1/1 -> Kp_phi/1
  Bus Selector/3 -> Sum3/2  "<P>"
  Bus Selector/4 -> Sum2/2  "<Q>"
  Kp_theta/1 -> Sum4/1
  theta_dot_r/1 -> Sum2/1
  Kp_phi/1 -> Sum5/1
  Sum2/1 -> Kd_theta/1
  Kd_theta/1 -> Sum4/2
  Sum4/1 -> tau_y/1
  phi_dot_r1/1 -> Sum3/1
  Sum3/1 -> Kd_phi/1
  Sum5/1 -> tau_x/1
  Kd_phi/1 -> Sum5/2

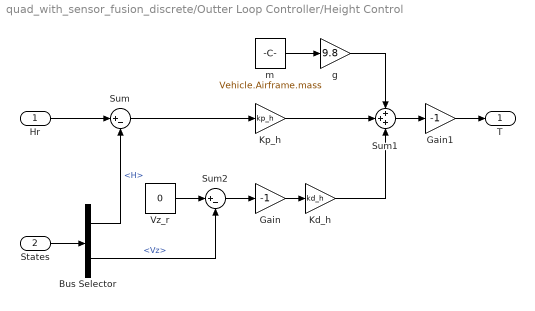
== system quad_with_sensor_fusion_discrete/Outter Loop Controller/Height Control ==
  Hr : Inport
  States : Inport  Port=2
  Bus Selector : BusSelector  OutputSignals=H,Vz
  Gain : Gain  Gain=-1
  Gain1 : Gain  Gain=-1
  Kd_h : Gain  Gain=kd_h
  Kp_h : Gain  Gain=kp_h
  Sum : Sum  Inputs=|+-
  Sum1 : Sum  Inputs=+++
  Sum2 : Sum  Inputs=|+-
  Vz_r : Constant  Value=0  SampleTime=0.005
  g : Gain  Gain=9.8
  m : Constant  Value=Vehicle.Airframe.mass  SampleTime=0.005
  T : Outport
  wires:
  Sum1/1 -> Gain1/1
  States/1 -> Bus Selector/1
  Hr/1 -> Sum/1
  Bus Selector/1 -> Sum/2  "<H>"
  Sum/1 -> Kp_h/1
  Kd_h/1 -> Sum1/3
  Bus Selector/2 -> Sum2/2  "<Vz>"
  m/1 -> g/1
  g/1 -> Sum1/1
  Sum2/1 -> Gain/1
  Kp_h/1 -> Sum1/2
  Gain/1 -> Kd_h/1
  Gain1/1 -> T/1
  Vz_r/1 -> Sum2/1

== system quad_with_sensor_fusion_discrete/Outter Loop Controller/Position Control ==
  xr : Inport
  yr : Inport  Port=2
  States : Inport  Port=3
  Bus Selector : BusSelector  OutputSignals=Y,X,ψ
  Kp_position : Gain  Gain=kp_position
  MATLAB Function : MATLAB Function  TreatAsAtomicUnit=on
  Mux : Mux  Inputs=2
  Sum : Sum  Inputs=|+-
  Sum1 : Sum  Inputs=|+-
  vxr : Outport
  vyr : Outport  Port=2
  wires:
  xr/1 -> Sum/1
  MATLAB Function/1(vxr) -> vxr/1  "vxr"
  MATLAB Function/2(vyr) -> vyr/1  "vyr"
  States/1 -> Bus Selector/1
  Bus Selector/3 -> MATLAB Function/2(psi)  "<ψ>"
  Bus Selector/2 -> Sum1/2  "<X>"
  Bus Selector/1 -> Sum/2  "<Y>"
  yr/1 -> Sum1/1
  Mux/1 -> Kp_position/1
  Sum1/1 -> Mux/2
  Kp_position/1 -> MATLAB Function/1(v)
  Sum/1 -> Mux/1

== system quad_with_sensor_fusion_discrete/Outter Loop Controller/Velocity Control ==
  vxr : Inport
  vyr : Inport  Port=2
  States : Inport  Port=3
  1 /g : Gain  Gain=1/9.8
  1/ g : Gain  Gain=1/9.8
  Bus Selector : BusSelector  OutputSignals=Vx,Vy
  Gain : Gain  Gain=-1
  Kp_vx : Gain  Gain=kp_vx
  Kp_vy : Gain  Gain=kp_vy
  Sum : Sum  Inputs=|+-
  Sum1 : Sum  Inputs=|+-
  theta_star : Outport
  phi_star : Outport  Port=2
  wires:
  vxr/1 -> Sum/1
  vyr/1 -> Sum1/1
  Sum/1 -> Gain/1
  1 /g/1 -> theta_star/1
  1/ g/1 -> phi_star/1
  Kp_vx/1 -> 1 /g/1
  Sum1/1 -> Kp_vy/1
  Kp_vy/1 -> 1/ g/1
  States/1 -> Bus Selector/1
  Bus Selector/1 -> Sum/2  "<Vx>"
  Bus Selector/2 -> Sum1/2  "<Vy>"
  Gain/1 -> Kp_vx/1

== system quad_with_sensor_fusion_discrete/Outter Loop Controller/Yaw Control ==
  Yawr : Inport
  States : Inport  Port=2
  Bus Selector : BusSelector  OutputSignals=ψ,R
  Kd_yaw : Gain  Gain=kd_yaw
  Kp_yaw : Gain  Gain=kp_yaw
  Sum : Sum  Inputs=|+-
  Sum1 : Sum  Inputs=|+-
  Sum2 : Sum  Inputs=|++
  Yaw_dot_r : Constant  Value=0  SampleTime=0.005
  tau_z : Outport
  wires:
  Sum2/1 -> tau_z/1
  Yawr/1 -> Sum/1
  Bus Selector/1 -> Sum/2  "<ψ>"
  Sum/1 -> Kp_yaw/1
  States/1 -> Bus Selector/1
  Bus Selector/2 -> Sum1/2  "<R>"
  Yaw_dot_r/1 -> Sum1/1
  Sum1/1 -> Kd_yaw/1
  Kp_yaw/1 -> Sum2/1
  Kd_yaw/1 -> Sum2/2

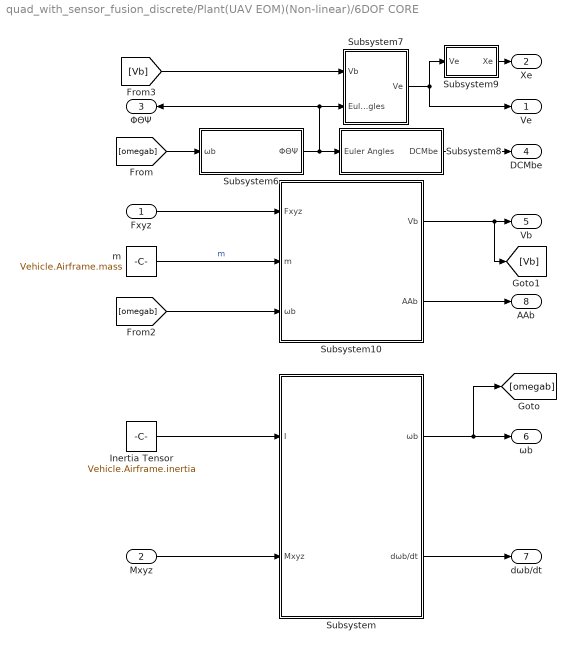
== system quad_with_sensor_fusion_discrete/Plant(UAV EOM)(Non-linear)/6DOF CORE ==
  Fxyz : Inport
  Mxyz : Inport  Port=2
  Inertia Tensor : Constant  Value=Vehicle.Airframe.inertia  VectorParams1D=off
  Subsystem : Subsystem
  Subsystem10 : Subsystem
  Subsystem6 : Subsystem
  Subsystem7 : Subsystem
      settings: PortSchema="{\"entries\":[{\"content\":{\"sides\":[{\"content\":{\"connectorIds\":[]},\"type\":\"ConnectorPlacement.EquallySpacedRectSide\",\"uuid\":\"1bd4c84a-8e3a-484f-b157-4fc2072173e9\"},{\"content\":{\"connectorIds\":[],\"side\":\"RIGHT\"},\"type\":\"ConnectorPlacement.EquallySpacedRectSide\",\"uuid\":\"5d02806b-ecd1-4a3d-b653-3060473a0baf\"},{\"content\":{\"connectorIds\":[\"Out1\"],\"side\":\"TOP\"},\"type\":\"ConnectorPlacement.EquallySpacedRectSide\",\"uuid\":\"b006a162-3e36-45b5-99bc-3480dd68e666\"},{\"content\":{\"connectorIds\":[\"In1\",\"In2\"],\"side\":\"BOTTOM\"},\"type\":\"ConnectorPlacement.EquallySpacedRectSide\",\"uuid\":\"a3921935-1893-4001-94f5-fd44c1c6a502\"},{\"content\":{\"connectorIds\":[],\"side\":\"HIDDEN\"},\"type\":\"ConnectorPlacement.EquallySpacedRectSide\",\"uuid\":\"8e011310-df3e-4a51-a6dd-e16af6e4adf7\"}]},\"type\":\"ConnectorPlacement.EquallySpacedConnector\",\"uuid\":\"87633363-c957-4eb9-bec4-3afb23cb2e66\"}],\"packageUris\":[\"http://schema.mathworks.com/mf0/Connector/R2020b\"],\"version\":\"1.0\"}"
  Subsystem8 : Subsystem
  Subsystem9 : Subsystem
  m : Constant  Value=Vehicle.Airframe.mass
  Ve : Outport
  Xe : Outport  Port=2
  ΦΘΨ : Outport  Port=3
  DCMbe : Outport  Port=4
  Vb : Outport  Port=5
  ωb : Outport  Port=6
  dωb/dt : Outport  Port=7
  AAb : Outport  Port=8
  wires:
  Subsystem9/1(Xe) -> Xe/1
  Subsystem8/1(DCMbe) -> DCMbe/1
  Subsystem7/1(Ve) -> Subsystem9/1(Ve), Ve/1
  Subsystem6/1(ΦΘΨ) -> Subsystem7/2(Euler Angles), ΦΘΨ/1, Subsystem8/1(Euler Angles)
  [omegab] -> Subsystem6/1(ωb)
  [Vb] -> Subsystem7/1(Vb)
  Subsystem10/1(Vb) -> [Vb], Vb/1
  Fxyz/1 -> Subsystem10/1(Fxyz)
  m/1 -> Subsystem10/2(m)  "m"
  [omegab] -> Subsystem10/3(ωb)
  Subsystem10/2(AAb) -> AAb/1
  Subsystem/1(ωb) -> [omegab], ωb/1
  Mxyz/1 -> Subsystem/2(Mxyz)
  Subsystem/2(dωb/dt) -> dωb/dt/1
  Inertia Tensor/1 -> Subsystem/1(I)

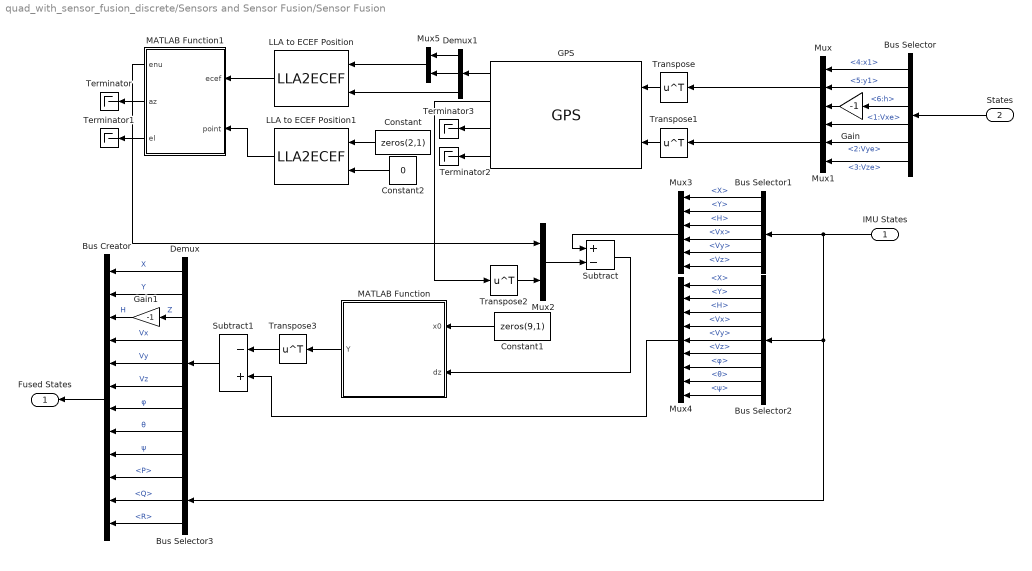
== system quad_with_sensor_fusion_discrete/Sensors and Sensor Fusion/Sensor Fusion ==
  IMU States : Inport
  States : Inport  Port=2
  Bus Creator : BusCreator  Inputs=12
  Bus Selector : BusSelector  OutputSignals=4:x1,5:y1,6:h,1:Vxe,2:Vye,3:Vze
  Bus Selector1 : BusSelector  OutputSignals=X,Y,H,Vx,Vy,Vz
  Bus Selector2 : BusSelector  OutputSignals=X,Y,H,Vx,Vy,Vz,φ,θ,ψ
  Bus Selector3 : BusSelector  OutputSignals=P,Q,R
  Constant : Constant  Value=zeros(2,1)  VectorParams1D=off  SampleTime=0.005
  Constant1 : Constant  Value=zeros(9,1)  VectorParams1D=off  SampleTime=0.005
  Constant2 : Constant  Value=0  SampleTime=0.005
  Demux : Demux  Outputs=9
  Demux1 : Demux  Outputs=3
  GPS : sensorgpslib/GPS  DispRefFrame=NED  PositionInputFormat=Local  ReferenceLocation=[ 0, 0, 0 ]  HorizontalPositionAccuracy=1.6  VerticalPositionAccuracy=3  VelocityAccuracy=0.1  DecayFactor=0.999  SeedDouble=67  SimulateUsing=Interpreted execution
      settings: LibrarySourceBlock=uavsimlib/GPS
  Gain : Gain  Gain=-1
  Gain1 : Gain  Gain=-1
  LLA to ECEF Position : LLA2ECEF
  LLA to ECEF Position1 : LLA2ECEF
  MATLAB Function : MATLAB Function  TreatAsAtomicUnit=on
  MATLAB Function1 : MATLAB Function  TreatAsAtomicUnit=on
  Mux : Mux  Inputs=3
  Mux1 : Mux  Inputs=3
  Mux2 : Mux  Inputs=2
  Mux3 : Mux  Inputs=6
  Mux4 : Mux  Inputs=9
  Mux5 : Mux  Inputs=2
  Subtract : Sum  Inputs=+-
  Subtract1 : Sum  Inputs=-+
  Terminator{,1..3} (4 alike) : Terminator
  Transpose{,1..3} (4 alike) : Math  Operator=transpose
  Fused States : Outport
  wires:
  States/1 -> Bus Selector/1
  GPS/1 -> Demux1/1
  GPS/4 -> Terminator2/1
  GPS/2 -> Transpose2/1
  GPS/3 -> Terminator3/1
  Bus Selector/2 -> Mux/2  "<5:y1>"
  Bus Selector/1 -> Mux/1  "<4:x1>"
  Bus Selector/3 -> Gain/1  "<6:h>"
  Bus Selector/5 -> Mux1/2  "<2:Vye>"
  Bus Selector/4 -> Mux1/1  "<1:Vxe>"
  Bus Selector/6 -> Mux1/3  "<3:Vze>"
  Gain/1 -> Mux/3
  IMU States/1 -> Bus Selector3/1, Bus Selector2/1, Bus Selector1/1
  MATLAB Function/1(Y) -> Transpose3/1
  MATLAB Function1/1(enu) -> Mux2/1
  Bus Selector1/1 -> Mux3/1  "<X>"
  Bus Selector1/2 -> Mux3/2  "<Y>"
  Bus Selector1/3 -> Mux3/3  "<H>"
  Bus Selector1/4 -> Mux3/4  "<Vx>"
  Bus Selector1/5 -> Mux3/5  "<Vy>"
  Bus Selector1/6 -> Mux3/6  "<Vz>"
  Mux2/1 -> Subtract/2
  Mux3/1 -> Subtract/1
  Subtract/1 -> MATLAB Function/2(dz)
  Mux4/1 -> Subtract1/2
  Bus Selector2/1 -> Mux4/1  "<X>"
  Bus Selector2/3 -> Mux4/3  "<H>"
  Bus Selector2/2 -> Mux4/2  "<Y>"
  Bus Selector2/4 -> Mux4/4  "<Vx>"
  Bus Selector2/5 -> Mux4/5  "<Vy>"
  Bus Selector2/6 -> Mux4/6  "<Vz>"
  Bus Selector2/7 -> Mux4/7  "<φ>"
  Bus Selector2/8 -> Mux4/8  "<θ>"
  Bus Selector2/9 -> Mux4/9  "<ψ>"
  Subtract1/1 -> Demux/1
  Bus Selector3/1 -> Bus Creator/10  "<P>"
  Bus Selector3/2 -> Bus Creator/11  "<Q>"
  Bus Selector3/3 -> Bus Creator/12  "<R>"
  Bus Creator/1 -> Fused States/1
  Demux/1 -> Bus Creator/1  "X"
  Demux/2 -> Bus Creator/2  "Y"
  Gain1/1 -> Bus Creator/3  "H"
  Demux/4 -> Bus Creator/4  "Vx"
  Demux/5 -> Bus Creator/5  "Vy"
  Demux/6 -> Bus Creator/6  "Vz"
  Demux/7 -> Bus Creator/7  "φ"
  Demux/8 -> Bus Creator/8  "θ"
  Demux/9 -> Bus Creator/9  "ψ"
  Demux/3 -> Gain1/1  "Z"
  Constant1/1 -> MATLAB Function/1(x0)
  LLA to ECEF Position/1 -> MATLAB Function1/1(ecef)
  Demux1/3 -> LLA to ECEF Position/2
  Demux1/1 -> Mux5/1
  Demux1/2 -> Mux5/2
  Mux5/1 -> LLA to ECEF Position/1
  MATLAB Function1/2(az) -> Terminator/1
  MATLAB Function1/3(el) -> Terminator1/1
  LLA to ECEF Position1/1 -> MATLAB Function1/2(point)
  Constant/1 -> LLA to ECEF Position1/1
  Constant2/1 -> LLA to ECEF Position1/2
  Transpose/1 -> GPS/1
  Transpose1/1 -> GPS/2
  Transpose2/1 -> Mux2/2
  Transpose3/1 -> Subtract1/1
  Mux/1 -> Transpose/1
  Mux1/1 -> Transpose1/1

== system quad_with_sensor_fusion_discrete/Sensors and Sensor Fusion/Subsystem6 ==
  ωb : Inport
  Demux : Demux  Outputs=3
  Discrete-Time Integrator : DiscreteIntegrator  IntegratorMethod=Integration: Trapezoidal  SampleTime=0.005  ICPrevOutput=DiscIntNeverNeededParam  ICPrevScaledInput=DiscIntNeverNeededParam
  Discrete-Time Integrator1 : DiscreteIntegrator  IntegratorMethod=Integration: Trapezoidal  SampleTime=0.005  ICPrevOutput=DiscIntNeverNeededParam  ICPrevScaledInput=DiscIntNeverNeededParam
  Discrete-Time Integrator2 : DiscreteIntegrator  IntegratorMethod=Integration: Trapezoidal  SampleTime=0.005  ICPrevOutput=DiscIntNeverNeededParam  ICPrevScaledInput=DiscIntNeverNeededParam
  MATLAB Function : MATLAB Function  TreatAsAtomicUnit=on
  MATLAB Function1 : MATLAB Function  TreatAsAtomicUnit=on
  MATLAB Function2 : MATLAB Function  TreatAsAtomicUnit=on
  Mux1 : Mux  Inputs=3
  ΦΘΨ : Outport
  wires:
  ωb/1 -> Demux/1
  Demux/1 -> MATLAB Function/1(P)
  Demux/2 -> MATLAB Function/2(Q), MATLAB Function2/1(Q), MATLAB Function1/1(Q)
  Demux/3 -> MATLAB Function/3(R), MATLAB Function2/2(R), MATLAB Function1/2(R)
  MATLAB Function/1(phidot) -> Discrete-Time Integrator/1  "dΦ/dt"
  Discrete-Time Integrator/1 -> Mux1/1, MATLAB Function2/3(phi), MATLAB Function1/3(phi), MATLAB Function/4(phi)  "Φ"
  Mux1/1 -> ΦΘΨ/1
  Discrete-Time Integrator1/1 -> Mux1/2, MATLAB Function2/4(theta), MATLAB Function/5(theta)  "Θ"
  MATLAB Function1/1(thetadot) -> Discrete-Time Integrator1/1  "dΘ/dt"
  Discrete-Time Integrator2/1 -> Mux1/3  "Ψ"
  MATLAB Function2/1(pusaidot) -> Discrete-Time Integrator2/1  "dΨ/dt"

== system quad_with_sensor_fusion_discrete/Sensors and Sensor Fusion/Vector to Bus ==
  In1 : Inport
  Bus Creator : BusCreator  Inputs=12
  Demux : Demux  Outputs=12
  Estimated States : Outport
  wires:
  Bus Creator/1 -> Estimated States/1
  In1/1 -> Demux/1
  Demux/12 -> Bus Creator/12  "ψ"
  Demux/11 -> Bus Creator/11  "θ"
  Demux/10 -> Bus Creator/10  "φ"
  Demux/9 -> Bus Creator/9  "R"
  Demux/8 -> Bus Creator/8  "Q"
  Demux/1 -> Bus Creator/1  "X"
  Demux/2 -> Bus Creator/2  "Y"
  Demux/3 -> Bus Creator/3  "H"
  Demux/4 -> Bus Creator/4  "Vx"
  Demux/5 -> Bus Creator/5  "Vy"
  Demux/6 -> Bus Creator/6  "Vz"
  Demux/7 -> Bus Creator/7  "P"

== system quad_with_sensor_fusion_discrete/Plant(UAV EOM)(Non-linear)/6DOF CORE/Subsystem ==
  I : Inport
  Mxyz : Inport  Port=2
  Discrete-Time Integrator : DiscreteIntegrator  IntegratorMethod=Integration: Trapezoidal  SampleTime=0.005  ICPrevOutput=DiscIntNeverNeededParam  ICPrevScaledInput=DiscIntNeverNeededParam
  Discrete-Time Integrator1 : DiscreteIntegrator  IntegratorMethod=Integration: Trapezoidal  SampleTime=0.005  ICPrevOutput=DiscIntNeverNeededParam  ICPrevScaledInput=DiscIntNeverNeededParam
  Discrete-Time Integrator2 : DiscreteIntegrator  IntegratorMethod=Integration: Trapezoidal  SampleTime=0.005  ICPrevOutput=DiscIntNeverNeededParam  ICPrevScaledInput=DiscIntNeverNeededParam
  MATLAB Function : MATLAB Function  TreatAsAtomicUnit=on
  Mux4 : Mux  Inputs=3
  Mux5 : Mux  Inputs=3
  ωb : Outport
  dωb/dt : Outport  Port=2
  wires:
  Discrete-Time Integrator1/1 -> Mux4/2  "Q"
  MATLAB Function/2(Q_dot) -> Discrete-Time Integrator1/1, Mux5/2  "dQ/dt"
  Discrete-Time Integrator/1 -> Mux4/1  "P"
  MATLAB Function/1(P_dot) -> Discrete-Time Integrator/1, Mux5/1  "dP/dt"
  MATLAB Function/3(R_dot) -> Discrete-Time Integrator2/1, Mux5/3  "dR/dt"
  Discrete-Time Integrator2/1 -> Mux4/3  "R"
  Mux5/1 -> dωb/dt/1
  Mxyz/1 -> MATLAB Function/2(M)
  I/1 -> MATLAB Function/1(I)
  Mux4/1 -> MATLAB Function/3(omega), ωb/1

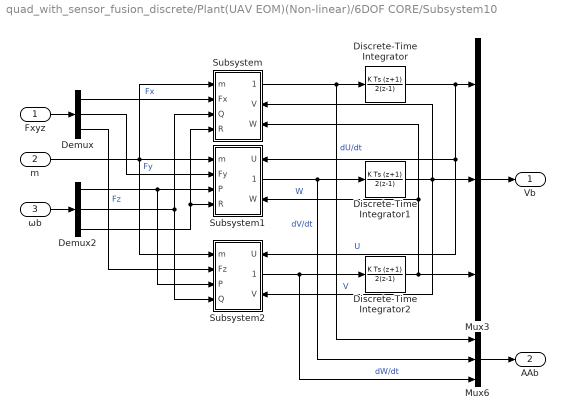
== system quad_with_sensor_fusion_discrete/Plant(UAV EOM)(Non-linear)/6DOF CORE/Subsystem10 ==
  Fxyz : Inport
  m : Inport  Port=2
  ωb : Inport  Port=3
  Demux : Demux  Outputs=3
  Demux2 : Demux  Outputs=3
  Discrete-Time Integrator : DiscreteIntegrator  IntegratorMethod=Integration: Trapezoidal  SampleTime=0.005  ICPrevOutput=DiscIntNeverNeededParam  ICPrevScaledInput=DiscIntNeverNeededParam
  Discrete-Time Integrator1 : DiscreteIntegrator  IntegratorMethod=Integration: Trapezoidal  SampleTime=0.005  ICPrevOutput=DiscIntNeverNeededParam  ICPrevScaledInput=DiscIntNeverNeededParam
  Discrete-Time Integrator2 : DiscreteIntegrator  IntegratorMethod=Integration: Trapezoidal  SampleTime=0.005  ICPrevOutput=DiscIntNeverNeededParam  ICPrevScaledInput=DiscIntNeverNeededParam
  Mux3 : Mux  Inputs=3
  Mux6 : Mux  Inputs=3
  Subsystem : Subsystem
      settings: PortSchema="{\"entries\":[{\"content\":{\"sides\":[{\"content\":{\"connectorIds\":[\"In1\",\"In2\",\"In3\",\"In4\"]},\"type\":\"ConnectorPlacement.EquallySpacedRectSide\",\"uuid\":\"326daed8-e070-42c4-b922-a1cfd1075610\"},{\"content\":{\"connectorIds\":[\"Out1\",\"In5\",\"In6\"],\"side\":\"RIGHT\"},\"type\":\"ConnectorPlacement.EquallySpacedRectSide\",\"uuid\":\"accd66e9-544e-4c99-a98b-e3a864bc5f81\"},{\"content\":{\"connectorIds\":[],\"side\":\"TOP\"},\"type\":\"ConnectorPlacement.EquallySpacedRectSide\",\"uuid\":\"83c3f4fc-532b-43a1-b874-56a52f4ca207\"},{\"content\":{\"connectorIds\":[],\"side\":\"HIDDEN\"},\"type\":\"ConnectorPlacement.EquallySpacedRectSide\",\"uuid\":\"414a66aa-d5b6-4143-97b4-f1301075a4c5\"}]},\"type\":\"ConnectorPlacement.EquallySpacedConnector\",\"uuid\":\"8a44064a-2e10-45f9-b0ec-d6ec6baf7018\"}],\"packageUris\":[\"http://schema.mathworks.com/mf0/Connector/R2020b\"],\"version\":\"1.0\"}"
  Subsystem1 : Subsystem
      settings: PortSchema="{\"entries\":[{\"content\":{\"sides\":[{\"content\":{\"connectorIds\":[\"In1\",\"In2\",\"In3\",\"In4\"]},\"type\":\"ConnectorPlacement.EquallySpacedRectSide\",\"uuid\":\"326daed8-e070-42c4-b922-a1cfd1075610\"},{\"content\":{\"connectorIds\":[\"In5\",\"Out1\",\"In6\"],\"side\":\"RIGHT\"},\"type\":\"ConnectorPlacement.EquallySpacedRectSide\",\"uuid\":\"accd66e9-544e-4c99-a98b-e3a864bc5f81\"},{\"content\":{\"connectorIds\":[],\"side\":\"TOP\"},\"type\":\"ConnectorPlacement.EquallySpacedRectSide\",\"uuid\":\"83c3f4fc-532b-43a1-b874-56a52f4ca207\"},{\"content\":{\"connectorIds\":[],\"side\":\"HIDDEN\"},\"type\":\"ConnectorPlacement.EquallySpacedRectSide\",\"uuid\":\"414a66aa-d5b6-4143-97b4-f1301075a4c5\"}]},\"type\":\"ConnectorPlacement.EquallySpacedConnector\",\"uuid\":\"8a44064a-2e10-45f9-b0ec-d6ec6baf7018\"}],\"packageUris\":[\"http://schema.mathworks.com/mf0/Connector/R2020b\"],\"version\":\"1.0\"}"
  Subsystem2 : Subsystem
      settings: PortSchema="{\"entries\":[{\"content\":{\"sides\":[{\"content\":{\"connectorIds\":[\"In1\",\"In2\",\"In3\",\"In4\"]},\"type\":\"ConnectorPlacement.EquallySpacedRectSide\",\"uuid\":\"326daed8-e070-42c4-b922-a1cfd1075610\"},{\"content\":{\"connectorIds\":[\"In5\",\"Out1\",\"In6\"],\"side\":\"RIGHT\"},\"type\":\"ConnectorPlacement.EquallySpacedRectSide\",\"uuid\":\"accd66e9-544e-4c99-a98b-e3a864bc5f81\"},{\"content\":{\"connectorIds\":[],\"side\":\"TOP\"},\"type\":\"ConnectorPlacement.EquallySpacedRectSide\",\"uuid\":\"83c3f4fc-532b-43a1-b874-56a52f4ca207\"},{\"content\":{\"connectorIds\":[],\"side\":\"HIDDEN\"},\"type\":\"ConnectorPlacement.EquallySpacedRectSide\",\"uuid\":\"414a66aa-d5b6-4143-97b4-f1301075a4c5\"}]},\"type\":\"ConnectorPlacement.EquallySpacedConnector\",\"uuid\":\"8a44064a-2e10-45f9-b0ec-d6ec6baf7018\"}],\"packageUris\":[\"http://schema.mathworks.com/mf0/Connector/R2020b\"],\"version\":\"1.0\"}"
  Vb : Outport
  AAb : Outport  Port=2
  wires:
  Subsystem2/1(dW/dt) -> Discrete-Time Integrator2/1, Mux6/3  "dW/dt"
  Demux2/3 -> Subsystem/4(R), Subsystem1/4(R)
  Demux/3 -> Subsystem2/2(Fz)  "Fz"
  Discrete-Time Integrator1/1 -> Mux3/2, Subsystem/5(V), Subsystem2/6(V)  "V"
  Subsystem/1(dU/dt) -> Discrete-Time Integrator/1, Mux6/1  "dU/dt"
  Subsystem1/1(dV/dt) -> Discrete-Time Integrator1/1, Mux6/2  "dV/dt"
  Demux2/1 -> Subsystem2/3(P), Subsystem1/3(P)
  Discrete-Time Integrator/1 -> Subsystem2/5(U), Subsystem1/5(U), Mux3/1  "U"
  Demux/1 -> Subsystem/2(Fx)  "Fx"
  m/1 -> Subsystem2/1(m), Subsystem/1(m), Subsystem1/1(m)
  Demux2/2 -> Subsystem/3(Q), Subsystem2/4(Q)
  Discrete-Time Integrator2/1 -> Subsystem1/6(W), Subsystem/6(W), Mux3/3  "W"
  Demux/2 -> Subsystem1/2(Fy)  "Fy"
  Mux6/1 -> AAb/1
  Fxyz/1 -> Demux/1
  Mux3/1 -> Vb/1
  ωb/1 -> Demux2/1

== system quad_with_sensor_fusion_discrete/Plant(UAV EOM)(Non-linear)/6DOF CORE/Subsystem6 ==
  ωb : Inport
  Demux : Demux  Outputs=3
  Discrete-Time Integrator : DiscreteIntegrator  IntegratorMethod=Integration: Trapezoidal  SampleTime=0.005  ICPrevOutput=DiscIntNeverNeededParam  ICPrevScaledInput=DiscIntNeverNeededParam
  Discrete-Time Integrator1 : DiscreteIntegrator  IntegratorMethod=Integration: Trapezoidal  SampleTime=0.005  ICPrevOutput=DiscIntNeverNeededParam  ICPrevScaledInput=DiscIntNeverNeededParam
  Discrete-Time Integrator2 : DiscreteIntegrator  IntegratorMethod=Integration: Trapezoidal  SampleTime=0.005  ICPrevOutput=DiscIntNeverNeededParam  ICPrevScaledInput=DiscIntNeverNeededParam
  MATLAB Function : MATLAB Function  TreatAsAtomicUnit=on
  MATLAB Function1 : MATLAB Function  TreatAsAtomicUnit=on
  MATLAB Function2 : MATLAB Function  TreatAsAtomicUnit=on
  Mux1 : Mux  Inputs=3
  ΦΘΨ : Outport
  wires:
  ωb/1 -> Demux/1
  Demux/1 -> MATLAB Function/1(P)
  Demux/2 -> MATLAB Function/2(Q), MATLAB Function2/1(Q), MATLAB Function1/1(Q)
  Demux/3 -> MATLAB Function/3(R), MATLAB Function2/2(R), MATLAB Function1/2(R)
  MATLAB Function/1(phidot) -> Discrete-Time Integrator/1  "dΦ/dt"
  Discrete-Time Integrator/1 -> Mux1/1, MATLAB Function2/3(phi), MATLAB Function1/3(phi), MATLAB Function/4(phi)  "Φ"
  Mux1/1 -> ΦΘΨ/1
  Discrete-Time Integrator1/1 -> Mux1/2, MATLAB Function2/4(theta), MATLAB Function/5(theta)  "Θ"
  MATLAB Function1/1(thetadot) -> Discrete-Time Integrator1/1  "dΘ/dt"
  Discrete-Time Integrator2/1 -> Mux1/3  "Ψ"
  MATLAB Function2/1(pusaidot) -> Discrete-Time Integrator2/1  "dΨ/dt"

== system quad_with_sensor_fusion_discrete/Plant(UAV EOM)(Non-linear)/6DOF CORE/Subsystem7 ==
  Vb : Inport
  Euler Angles : Inport  Port=2
  Mux : Mux  Inputs=3
  Subsystem : Subsystem
  Subsystem1 : Subsystem
  Subsystem2 : Subsystem
  Ve : Outport
  wires:
  Mux/1 -> Ve/1
  Euler Angles/1 -> Subsystem/2(Euler Angles), Subsystem1/2(Euler Angles), Subsystem2/2(Euler Angles)
  Vb/1 -> Subsystem/1(Vb), Subsystem2/1(Vb), Subsystem1/1(Vb)
  Subsystem/1(Vxe) -> Mux/1
  Subsystem1/1(Vye) -> Mux/2
  Subsystem2/1(Vze) -> Mux/3

== system quad_with_sensor_fusion_discrete/Plant(UAV EOM)(Non-linear)/6DOF CORE/Subsystem8 ==
  Euler Angles : Inport
  MATLAB Function : MATLAB Function  TreatAsAtomicUnit=on
  DCMbe : Outport
  wires:
  MATLAB Function/1(y) -> DCMbe/1
  Euler Angles/1 -> MATLAB Function/1(u)

== system quad_with_sensor_fusion_discrete/Plant(UAV EOM)(Non-linear)/6DOF CORE/Subsystem9 ==
  Ve : Inport
  Demux3 : Demux  Outputs=3
  Discrete-Time Integrator : DiscreteIntegrator  IntegratorMethod=Integration: Trapezoidal  SampleTime=0.005  ICPrevOutput=DiscIntNeverNeededParam  ICPrevScaledInput=DiscIntNeverNeededParam
  Discrete-Time Integrator1 : DiscreteIntegrator  IntegratorMethod=Integration: Trapezoidal  SampleTime=0.005  ICPrevOutput=DiscIntNeverNeededParam  ICPrevScaledInput=DiscIntNeverNeededParam
  Discrete-Time Integrator2 : DiscreteIntegrator  IntegratorMethod=Integration: Trapezoidal  InitialCondition=-10  SampleTime=0.005  ICPrevOutput=DiscIntNeverNeededParam  ICPrevScaledInput=DiscIntNeverNeededParam
  Mux1 : Mux  Inputs=3
  Xe : Outport
  wires:
  Discrete-Time Integrator/1 -> Mux1/1  "Xe"
  Discrete-Time Integrator2/1 -> Mux1/3  "Ze"
  Demux3/3 -> Discrete-Time Integrator2/1
  Demux3/2 -> Discrete-Time Integrator1/1
  Discrete-Time Integrator1/1 -> Mux1/2  "Ye"
  Demux3/1 -> Discrete-Time Integrator/1
  Ve/1 -> Demux3/1
  Mux1/1 -> Xe/1

== system quad_with_sensor_fusion_discrete/Plant(UAV EOM)(Non-linear)/6DOF CORE/Subsystem10/Subsystem ==
  m : Inport
  Fx : Inport  Port=2
  Q : Inport  Port=3
  R : Inport  Port=4
  V : Inport  Port=5
  W : Inport  Port=6
  MATLAB Function : MATLAB Function  TreatAsAtomicUnit=on
  dU/dt : Outport
  wires:
  m/1 -> MATLAB Function/1(m)
  Fx/1 -> MATLAB Function/2(Fx)
  V/1 -> MATLAB Function/3(V)
  W/1 -> MATLAB Function/4(W)
  Q/1 -> MATLAB Function/5(Q)
  R/1 -> MATLAB Function/6(R)
  MATLAB Function/1(udot) -> dU/dt/1

== system quad_with_sensor_fusion_discrete/Plant(UAV EOM)(Non-linear)/6DOF CORE/Subsystem10/Subsystem1 ==
  m : Inport
  Fy : Inport  Port=2
  P : Inport  Port=3
  R : Inport  Port=4
  U : Inport  Port=5
  W : Inport  Port=6
  MATLAB Function : MATLAB Function  TreatAsAtomicUnit=on
  dV/dt : Outport
  wires:
  m/1 -> MATLAB Function/1(m)
  Fy/1 -> MATLAB Function/2(Fy)
  U/1 -> MATLAB Function/3(U)
  W/1 -> MATLAB Function/4(W)
  P/1 -> MATLAB Function/5(P)
  R/1 -> MATLAB Function/6(R)
  MATLAB Function/1(vdot) -> dV/dt/1

== system quad_with_sensor_fusion_discrete/Plant(UAV EOM)(Non-linear)/6DOF CORE/Subsystem10/Subsystem2 ==
  m : Inport
  Fz : Inport  Port=2
  P : Inport  Port=3
  Q : Inport  Port=4
  U : Inport  Port=5
  V : Inport  Port=6
  MATLAB Function : MATLAB Function  TreatAsAtomicUnit=on
  dW/dt : Outport
  wires:
  m/1 -> MATLAB Function/1(m)
  Fz/1 -> MATLAB Function/2(Fz)
  U/1 -> MATLAB Function/3(U)
  V/1 -> MATLAB Function/4(V)
  P/1 -> MATLAB Function/5(P)
  Q/1 -> MATLAB Function/6(Q)
  MATLAB Function/1(wdot) -> dW/dt/1

== system quad_with_sensor_fusion_discrete/Plant(UAV EOM)(Non-linear)/6DOF CORE/Subsystem7/Subsystem ==
  Vb : Inport
  Euler Angles : Inport  Port=2
  Demux : Demux  Outputs=3
  Demux1 : Demux  Outputs=3
  MATLAB Function : MATLAB Function  TreatAsAtomicUnit=on
  Vxe : Outport
  wires:
  Euler Angles/1 -> Demux1/1
  Vb/1 -> Demux/1
  Demux/1 -> MATLAB Function/1(U)
  Demux/2 -> MATLAB Function/2(V)
  Demux/3 -> MATLAB Function/3(W)
  Demux1/1 -> MATLAB Function/4(phi)
  Demux1/2 -> MATLAB Function/5(theta)
  Demux1/3 -> MATLAB Function/6(pusai)
  MATLAB Function/1(Vxe) -> Vxe/1

== system quad_with_sensor_fusion_discrete/Plant(UAV EOM)(Non-linear)/6DOF CORE/Subsystem7/Subsystem1 ==
  Vb : Inport
  Euler Angles : Inport  Port=2
  Demux : Demux  Outputs=3
  Demux1 : Demux  Outputs=3
  MATLAB Function : MATLAB Function  TreatAsAtomicUnit=on
  Vye : Outport
  wires:
  Euler Angles/1 -> Demux1/1
  Vb/1 -> Demux/1
  Demux/1 -> MATLAB Function/1(U)
  Demux/2 -> MATLAB Function/2(V)
  Demux/3 -> MATLAB Function/3(W)
  Demux1/1 -> MATLAB Function/4(phi)
  Demux1/2 -> MATLAB Function/5(theta)
  Demux1/3 -> MATLAB Function/6(pusai)
  MATLAB Function/1(Vye) -> Vye/1

== system quad_with_sensor_fusion_discrete/Plant(UAV EOM)(Non-linear)/6DOF CORE/Subsystem7/Subsystem2 ==
  Vb : Inport
  Euler Angles : Inport  Port=2
  Demux : Demux  Outputs=3
  Demux1 : Demux  Outputs=3
  MATLAB Function : MATLAB Function  TreatAsAtomicUnit=on
  Terminator : Terminator
  Vze : Outport
  wires:
  Euler Angles/1 -> Demux1/1
  Vb/1 -> Demux/1
  Demux/1 -> MATLAB Function/1(U)
  Demux/2 -> MATLAB Function/2(V)
  Demux/3 -> MATLAB Function/3(W)
  Demux1/1 -> MATLAB Function/4(phi)
  Demux1/2 -> MATLAB Function/5(theta)
  Demux1/3 -> Terminator/1
  MATLAB Function/1(Vze) -> Vze/1

== matlab function quad_with_sensor_fusion_discrete/Sensors and Sensor Fusion/Sensor Fusion/MATLAB Function ==
  data: x0 input; Y output; dz input
function Y = DPVKF_lc(x0,dz)
    sigma_h = 1.6;
    sigma_v = 3;
    sigma_velocity = 0.1;
    sigma_a = 0.01;
    sigma_omega = 0.001;
    delta_t = 1/200;

    Q = diag([zeros(3,1); ...
              1/delta_t*sigma_a^2*ones(3,1); ...
              1/delta_t*sigma_omega^2*ones(3,1)]);
    Phi = eye(9);
    Phi(1,4) = delta_t;
    Phi(2,5) = delta_t;
    Phi(3,6) = delta_t;
    Phi(1,4) = delta_t;
    Phi(2,5) = delta_t;
    Phi(3,6) = delta_t;
    H = eye(6);
    H = [H,zeros(6,3)];

    Gamma = diag([zeros(3,1);delta_t*ones(6,1)]);
    x = zeros(9,1);
%     K = zeros(9,6);
    P = diag(1e0*ones(9,1));
%     Y = zeros(9,1);

    a = 1/delta_t;
    R = diag([sigma_h^2+a*sigma_a^2; ...
              sigma_h^2+a*sigma_a^2; ...
              sigma_v^2+a*sigma_a^2; ...
             (sigma_velocity^2+a*sigma_a^2)*ones(3,1)]);
    P = Phi*P*Phi'+Gamma*Q*Gamma';
    K = (P*H')*inv(H*P*H'+R);
    x = x+K*(dz-H*x);
    Y = x;
end

== matlab function quad_with_sensor_fusion_discrete/Sensors and Sensor Fusion/Sensor Fusion/MATLAB Function1 ==
  data: ecef input; enu output; point input; az output; el output
function [enu,az,el] = ECEF2ENU(ecef,point)
%% ECEF2ENU 此处提供此函数的摘要
% ecef: Target Coordinate in ECEF
% point: ENU's Origin Coordinate in LLA
%%   此处提供详细说明
    phi = point(1)*pi/180;
    lambda = point(2)*pi/180;
    ecef_diff = ecef-point;
    A = [-sin(lambda),cos(lambda),0;
        -cos(lambda)*sin(phi),-sin(lambda)*sin(phi),cos(phi);
        cos(lambda)*cos(phi),sin(lambda)*cos(phi),sin(phi)];
    enu = A*ecef_diff;
    
    if(enu(2)>=0)
        az = atan(enu(1)/enu(2));
    else
        az = pi+atan(enu(1)/enu(2));
    end
    el = asin(enu(3)/norm(enu));
end
